simulink model "CS637Assignment1_1_1"  (R2022a)
settings: Solver=VariableStepAuto  StartTime=0.0  StopTime=10.0  RelTol=1e-3
settings Model: Creator=kaush  LastModifiedBy=kaush

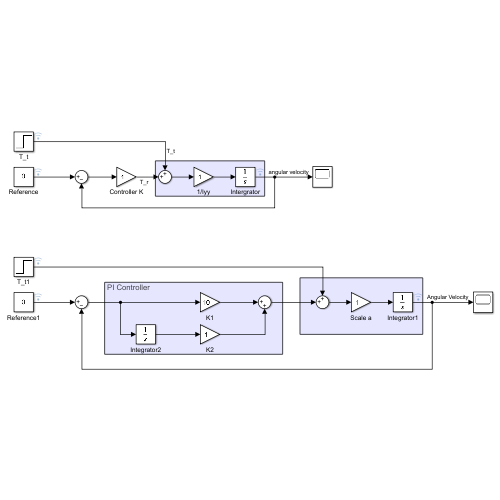
[thumbnail: Simulink's stored preview of the top-level diagram]
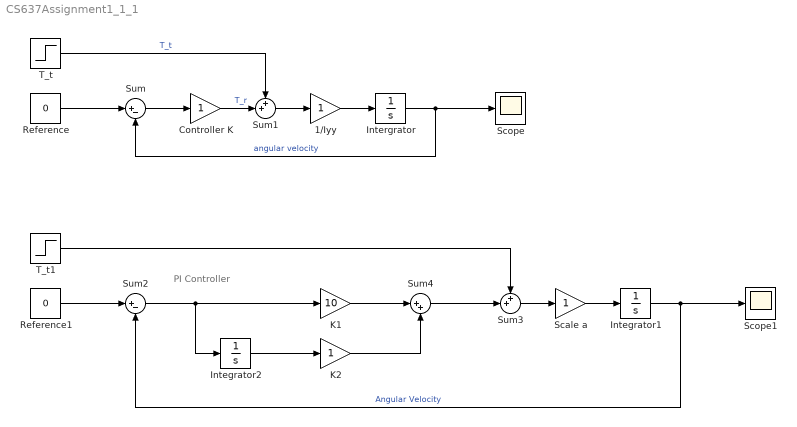
== system CS637Assignment1_1_1 ==
  note: PI Controller
  1/Iyy : Gain
  Controller K : Gain
  Integrator1 : Integrator
  Integrator2 : Integrator
  Intergrator : Integrator
  K1 : Gain  Gain=10
  K2 : Gain
  Reference : Constant  Value=0
  Reference1 : Constant  Value=0
  Scale a : Gain
  Scope : Scope
  Scope1 : Scope
  Sum : Sum  Inputs=|+-
  Sum1 : Sum  Inputs=++|
  Sum2 : Sum  Inputs=|+-
  Sum3 : Sum  Inputs=++|
  Sum4 : Sum  Inputs=|++
  T_t : Step  Time=0  After=0.5  SampleTime=0
  T_t1 : Step  Time=0  After=0.5  SampleTime=0
  wires:
  Reference/1 -> Sum/1
  Sum/1 -> Controller K/1
  Sum1/1 -> 1/Iyy/1
  1/Iyy/1 -> Intergrator/1
  Intergrator/1 -> Sum/2, Scope/1  "angular velocity"
  T_t/1 -> Sum1/1  "T_t"
  Scale a/1 -> Integrator1/1
  Sum3/1 -> Scale a/1
  Integrator1/1 -> Sum2/2, Scope1/1  "Angular Velocity"
  Reference1/1 -> Sum2/1
  Sum2/1 -> K1/1, Integrator2/1
  K2/1 -> Sum4/2
  Integrator2/1 -> K2/1
  K1/1 -> Sum4/1
  Controller K/1 -> Sum1/2  "T_r"
  T_t1/1 -> Sum3/1
  Sum4/1 -> Sum3/2
